simulink model "d_006"  (Simulink 9.3)
settings: Solver=ode45  StartTime=0.0  StopTime=10.0  RelTol=1e-3  EnableMultiTasking=on
settings Model: Creator=fmilano  LastModifiedBy=fmilano  ExtModeAutoUpdateStatusClock=off
settings DataIOCC: LimitDataPoints=on
settings OptimizationCC: BooleanDataType=off  InitFltsAndDblsToZero=on  LifeSpan=auto
settings DebuggingCC: SaveWithParameterizedLinksMsg=none  SignalResolutionControl=TryResolveAllWithWarning  MultiTaskDSMMsg=warning  MultiTaskCondExecSysMsg=none  FcnCallInpInsideContextMsg=error  SFUnexpectedBacktrackingDiag=error  SFNoUnconditionalDefaultTransitionDiag=error  SFExecutionAtInitializationDiag=warning  ArithmeticOperatorsInVariantConditions=error
settings HardwareCC: ProdBitPerPointer=64  ProdBitPerSizeT=64  ProdBitPerPtrDiffT=64  ProdLargestAtomicFloat=Float  ProdIntDivRoundTo=Zero  ProdEndianess=LittleEndian  ProdWordSize=64  ProdHWDeviceType=Intel->x86-64 (Windows64)  TargetUnknown=on
settings SFSimCC: SimUseLocalCustomCode=on
settings RTWCC: RTWUseLocalCustomCode=on
settings CodeAppCC: StateflowObjectComments=off
settings GRTTargetCC: TargetFcnLib=ansi_tfl_tmw.mat  TargetLangStandard=C99 (ISO)  CodeReplacementLibrary=ANSI_C  ParMdlRefBuildCompliant=off  CompOptLevelCompliant=off  CPPClassGenCompliant=off
settings ConfigComp: CovExternalEMLEnable=on

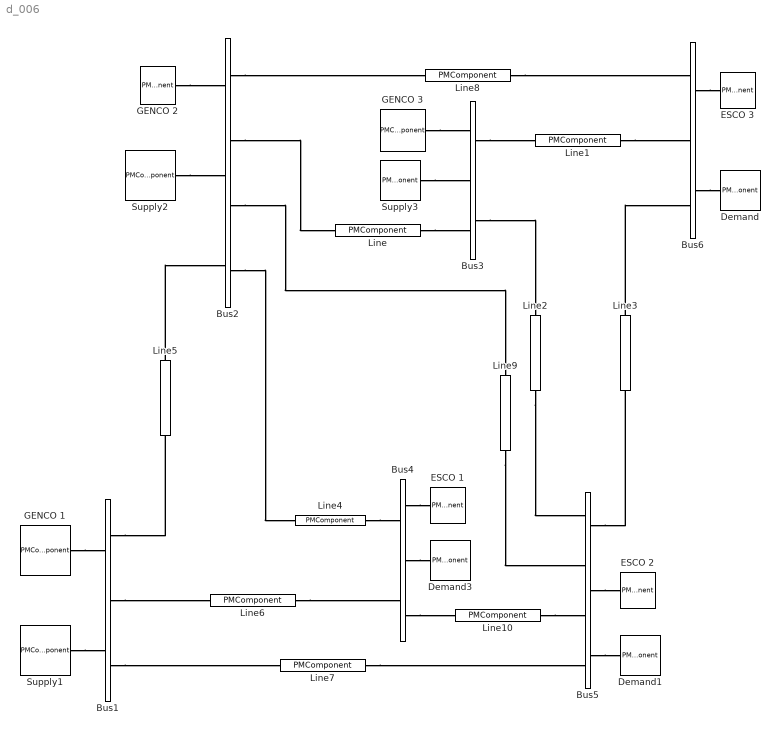
== system d_006 ==
  Bus1 : PMComponent  Tag=PSATblock  Description=Connection  PhysicalDomain=psatdomain  LeftPortType=p1  RightPortType=p1  LConnTagsString=__newl0|__newl1  RConnTagsString=__newr0|__newr1|__newr2  mask(Bus){in=2, out=3, p2q=400, p3_4q=[1.00   0.00], p5q=2, p6q=1}
      mask prompts: in "Number of inputs:"; out "Number of outputs:"; p2q "Voltage Rating [kV]"; p3_4q "Voltage initial guess [p.u.  rad]"; p5q "Area number"; p6q "Region number"
      mask help: Bus block.
      mask init:
      | fm_inout
      mask Callback p5q: fm_block
      mask Display: plot([0 1 1 0 0],[0 0 1 1 0])
  Bus2 : PMComponent  Tag=PSATblock  Description=Connection  PhysicalDomain=psatdomain  LeftPortType=p1  RightPortType=p1  LConnTagsString=__newl0|__newl1|__newl2  RConnTagsString=__newr0|__newr1|__newr2|__newr3  mask(Bus){in=3, out=4, p2q=400, p3_4q=[1.00   0.00], p5q=2, p6q=1}
      mask prompts: in "Number of inputs:"; out "Number of outputs:"; p2q "Voltage Rating [kV]"; p3_4q "Voltage initial guess [p.u.  rad]"; p5q "Area number"; p6q "Region number"
      mask help: Bus block.
      mask init:
      | fm_inout
      mask Callback p5q: fm_block
      mask Display: plot([0 1 1 0 0],[0 0 1 1 0])
  Bus3 : PMComponent  Tag=PSATblock  Description=Connection  PhysicalDomain=psatdomain  LeftPortType=p1  RightPortType=p1  LConnTagsString=__newl0|__newl1|__newl2  RConnTagsString=__newr0|__newr1  mask(Bus){in=3, out=2, p2q=400, p3_4q=[1.00   0.00], p5q=2, p6q=1}
      mask prompts: in "Number of inputs:"; out "Number of outputs:"; p2q "Voltage Rating [kV]"; p3_4q "Voltage initial guess [p.u.  rad]"; p5q "Area number"; p6q "Region number"
      mask help: Bus block.
      mask init:
      | fm_inout
      mask Callback p5q: fm_block
      mask Display: plot([0 1 1 0 0],[0 0 1 1 0])
  Bus4 : PMComponent  Tag=PSATblock  Description=Connection  PhysicalDomain=psatdomain  LeftPortType=p1  RightPortType=p1  LConnTagsString=__newl0|__newl1  RConnTagsString=__newr0|__newr1|__newr2  mask(Bus){in=2, out=3, p2q=400, p3_4q=[1.00   0.00], p5q=2, p6q=1}
      mask prompts: in "Number of inputs:"; out "Number of outputs:"; p2q "Voltage Rating [kV]"; p3_4q "Voltage initial guess [p.u.  rad]"; p5q "Area number"; p6q "Region number"
      mask help: Bus block.
      mask init:
      | fm_inout
      mask Callback p5q: fm_block
      mask Display: plot([0 1 1 0 0],[0 0 1 1 0])
  Bus5 : PMComponent  Tag=PSATblock  Description=Connection  PhysicalDomain=psatdomain  LeftPortType=p1  RightPortType=p1  LConnTagsString=__newl0|__newl1|__newl2|__newl3  RConnTagsString=__newr0|__newr1|__newr2  mask(Bus){in=4, out=3, p2q=400, p3_4q=[1.00   0.00], p5q=2, p6q=1}
      mask prompts: in "Number of inputs:"; out "Number of outputs:"; p2q "Voltage Rating [kV]"; p3_4q "Voltage initial guess [p.u.  rad]"; p5q "Area number"; p6q "Region number"
      mask help: Bus block.
      mask init:
      | fm_inout
      mask Callback p5q: fm_block
      mask Display: plot([0 1 1 0 0],[0 0 1 1 0])
  Bus6 : PMComponent  Tag=PSATblock  Description=Connection  PhysicalDomain=psatdomain  LeftPortType=p1  RightPortType=p1  LConnTagsString=__newl0|__newl1|__newl2  RConnTagsString=__newr0|__newr1  mask(Bus){in=3, out=2, p2q=400, p3_4q=[1.00   0.00], p5q=2, p6q=1}
      mask prompts: in "Number of inputs:"; out "Number of outputs:"; p2q "Voltage Rating [kV]"; p3_4q "Voltage initial guess [p.u.  rad]"; p5q "Area number"; p6q "Region number"
      mask help: Bus block.
      mask init:
      | fm_inout
      mask Callback p5q: fm_block
      mask Display: plot([0 1 1 0 0],[0 0 1 1 0])
  Demand : PMComponent  Tag=PSATblock  Description=OPF & CPF  PhysicalDomain=psatdomain  LeftPortType=p1  RightPortType=p1  LConnTagsString=__newl0  mask(Demand){p2q=100, p3q=0.2, p4q=0.66666*0.1, p5_6q=[0.2  0.00001], p8_9_10q=[0.00  9.5  0.00], p11_12_13q=[0.00  0.00  0.00], p14q=off, p15q=0, p16_17q=[0 0], out=0, p18q=on}
      mask prompts: p2q "Power Rating [MVA]"; p3q "Active Power [p.u.]"; p4q "Reactive Power [p.u.]"; p5_6q "Max and Min Power Demand [p.u.  p.u.]"; p8_9_10q "Cost = a + b*P + c*P^2 [$/h, $/MWh, $/(MW)^2 h]"; p11_12_13q "Cost = a + b*Q + c*Q^2 [$/h, $/MVArh, $/(MVAr)^2 h]"; p14q "Allow Unit Commitment"; p15q "Tie Breaking Cost [$/h]"; p16_17q "Up and down congestion costs [$/h $/h]"; out "Number of Output Signals"; p18q "Connected"
      mask help: This block defines a constant power load for bifurcation and market studies.
      mask init:
      | fm_inout;
      | [xs,ys]=fm_draw('$');
      mask TypeOptions out: 0 | 1
      mask Callback p18q: fm_block
      mask Display:
      | plot([ 1.0000    -0.5   -0.5  1],[ 0    0.866    -0.866    0])
      | color('blue')
      | plot(0.6*xs,0.6*ys)
  Demand1 : PMComponent  Tag=PSATblock  Description=OPF & CPF  PhysicalDomain=psatdomain  LeftPortType=p1  RightPortType=p1  LConnTagsString=__newl0  mask(Demand){p2q=100, p3q=0.1, p4q=0.7*0.1, p5_6q=[0.1  0.00001], p8_9_10q=[0.00  10.5  0.00], p11_12_13q=[0.00  0.00  0.00], p14q=off, p15q=0, p16_17q=[0 0], out=0, p18q=on}
      mask prompts: p2q "Power Rating [MVA]"; p3q "Active Power [p.u.]"; p4q "Reactive Power [p.u.]"; p5_6q "Max and Min Power Demand [p.u.  p.u.]"; p8_9_10q "Cost = a + b*P + c*P^2 [$/h, $/MWh, $/(MW)^2 h]"; p11_12_13q "Cost = a + b*Q + c*Q^2 [$/h, $/MVArh, $/(MVAr)^2 h]"; p14q "Allow Unit Commitment"; p15q "Tie Breaking Cost [$/h]"; p16_17q "Up and down congestion costs [$/h $/h]"; out "Number of Output Signals"; p18q "Connected"
      mask help: This block defines a constant power load for bifurcation and market studies.
      mask init:
      | fm_inout;
      | [xs,ys]=fm_draw('$');
      mask TypeOptions out: 0 | 1
      mask Callback p18q: fm_block
      mask Display:
      | plot([ 1.0000    -0.5   -0.5  1],[ 0    0.866    -0.866    0])
      | color('blue')
      | plot(0.6*xs,0.6*ys)
  Demand3 : PMComponent  Tag=PSATblock  Description=OPF & CPF  PhysicalDomain=psatdomain  LeftPortType=p1  RightPortType=p1  LConnTagsString=__newl0  mask(Demand){p2q=100, p3q=0.25, p4q=0.66666*0.25, p5_6q=[0.25  0.00001], p8_9_10q=[0.00  12  0.00], p11_12_13q=[0.00  0.00  0.00], p14q=off, p15q=0, p16_17q=[0 0], out=0, p18q=on}
      mask prompts: p2q "Power Rating [MVA]"; p3q "Active Power [p.u.]"; p4q "Reactive Power [p.u.]"; p5_6q "Max and Min Power Demand [p.u.  p.u.]"; p8_9_10q "Cost = a + b*P + c*P^2 [$/h, $/MWh, $/(MW)^2 h]"; p11_12_13q "Cost = a + b*Q + c*Q^2 [$/h, $/MVArh, $/(MVAr)^2 h]"; p14q "Allow Unit Commitment"; p15q "Tie Breaking Cost [$/h]"; p16_17q "Up and down congestion costs [$/h $/h]"; out "Number of Output Signals"; p18q "Connected"
      mask help: This block defines a constant power load for bifurcation and market studies.
      mask init:
      | fm_inout;
      | [xs,ys]=fm_draw('$');
      mask TypeOptions out: 0 | 1
      mask Callback p18q: fm_block
      mask Display:
      | plot([ 1.0000    -0.5   -0.5  1],[ 0    0.866    -0.866    0])
      | color('blue')
      | plot(0.6*xs,0.6*ys)
  ESCO 1 : PMComponent  Tag=PSATblock  Description=Power Flow  PhysicalDomain=psatdomain  LeftPortType=p1  RightPortType=p1  LConnTagsString=__newl0  mask(PQ){p2_3q=[100  400], p4_5q=[0.90  0.60], p6_7q=[1.1  0.9], p8q=off, p9q=on}
      mask prompts: p2_3q "Power and Voltage Ratings [MVA, kV]"; p4_5q "Active and Reactive Powers [p.u.  p.u.]"; p6_7q "Maximum and Minimum Allowable Voltage [p.u.   p.u.]"; p8q "Allow conversion to impendance for min & max voltage"; p9q "Connected"
      mask help:
      | This block defines a constant power load:
      |
      | P = Pcost.
      | Q = Qcost.
      mask Callback p8q: fm_block
      mask Callback p9q: fm_block
      mask Display: plot([1 -0.5 -0.5 1],[0 0.866 -0.866 0])
  ESCO 2 : PMComponent  Tag=PSATblock  Description=Power Flow  PhysicalDomain=psatdomain  LeftPortType=p1  RightPortType=p1  LConnTagsString=__newl0  mask(PQ){p2_3q=[100  400], p4_5q=[1.00  0.70], p6_7q=[1.1  0.9], p8q=off, p9q=on}
      mask prompts: p2_3q "Power and Voltage Ratings [MVA, kV]"; p4_5q "Active and Reactive Powers [p.u.  p.u.]"; p6_7q "Maximum and Minimum Allowable Voltage [p.u.   p.u.]"; p8q "Allow conversion to impendance for min & max voltage"; p9q "Connected"
      mask help:
      | This block defines a constant power load:
      |
      | P = Pcost.
      | Q = Qcost.
      mask Callback p8q: fm_block
      mask Callback p9q: fm_block
      mask Display: plot([1 -0.5 -0.5 1],[0 0.866 -0.866 0])
  ESCO 3 : PMComponent  Tag=PSATblock  Description=Power Flow  PhysicalDomain=psatdomain  LeftPortType=p1  RightPortType=p1  LConnTagsString=__newl0  mask(PQ){p2_3q=[100  400], p4_5q=[0.90  0.60], p6_7q=[1.1  0.9], p8q=off, p9q=on}
      mask prompts: p2_3q "Power and Voltage Ratings [MVA, kV]"; p4_5q "Active and Reactive Powers [p.u.  p.u.]"; p6_7q "Maximum and Minimum Allowable Voltage [p.u.   p.u.]"; p8q "Allow conversion to impendance for min & max voltage"; p9q "Connected"
      mask help:
      | This block defines a constant power load:
      |
      | P = Pcost.
      | Q = Qcost.
      mask Callback p8q: fm_block
      mask Callback p9q: fm_block
      mask Display: plot([1 -0.5 -0.5 1],[0 0.866 -0.866 0])
  GENCO 1 : PMComponent  Tag=PSATblock  Description=Power Flow  PhysicalDomain=psatdomain  LeftPortType=p1  RightPortType=p1  RConnTagsString=__newr0  mask(PV){p2_3q=[100  400], p4q=0.9, p5q=1.05, p6_7q=[1.5  -1.5], p8_9q=[1.1  0.9], p10q=1, p11q=on}
      mask prompts: p2_3q "Power and Voltage Ratings [MVA, kV]"; p4q "Active Power [p.u.]"; p5q "Voltage Magnitude [p.u.]"; p6_7q "Qmax & Qmin [p.u.  p.u.]"; p8_9q "Vmax & Vmin [p.u.  p.u.]"; p10q "Loss Participation Factor"; p11q "Connected"
      mask help:
      | This block defines a PV bus for load flow studies:
      |
      | P = Pcost.
      | V = Vdes.
      mask init:
      | [x,y] = fm_draw('circle');
      | [xp,yp] = fm_draw('P');
      mask Callback p11q: fm_block
      mask Display:
      | plot(x,y)
      | color('blue')
      | plot(0.3*xp-0.35,0.6*yp,[0.1 0.3 0.5],[0.3 -0.3 0.3])
  GENCO 2 : PMComponent  Tag=PSATblock  Description=Power Flow  PhysicalDomain=psatdomain  LeftPortType=p1  RightPortType=p1  RConnTagsString=__newr0  mask(SW){p2_3q=[100  400], p4q=1.05, p5q=0.00, p6_7q=[1.5  -1.5], p8_9q=[1.1  0.9], p10q=1.4, p11q=1, p12q=on, p13q=on}
      mask prompts: p2_3q "Power and Voltage Ratings [MVA, kV]"; p4q "Voltage Magnitude [p.u.]"; p5q "Reference Phase Angle [rad]"; p6_7q "Qmax and Qmin [p.u.  p.u.]"; p8_9q "Vmax and Vmin  [p.u.  p.u.]"; p10q "Active Power Guess [p.u.]"; p11q "Loss Participation Factor"; p12q "Reference bus"; p13q "Connected"
      mask help:
      | This block defines a V-theta bus:
      |
      | V = V_des
      | theta = theta_des
      mask init:
      | [x,y] = fm_draw('circle');
      | [xt,yt] = fm_draw('theta');
      mask Callback p12q: fm_block
      mask Callback p13q: fm_block
      mask Display: plot([0 1 1 0 0],[0 0 1 1 0]), color('blue'), plot([0 1],[0 1],[0 1],[1 0],[0.5 1 0.5 0 0.5],[0 0.5 1 0.5 0])
  GENCO 3 : PMComponent  Tag=PSATblock  Description=Power Flow  PhysicalDomain=psatdomain  LeftPortType=p1  RightPortType=p1  RConnTagsString=__newr0  mask(PV){p2_3q=[100  400], p4q=0.6, p5q=1.05, p6_7q=[1.5  -1.5], p8_9q=[1.1  0.9], p10q=1, p11q=on}
      mask prompts: p2_3q "Power and Voltage Ratings [MVA, kV]"; p4q "Active Power [p.u.]"; p5q "Voltage Magnitude [p.u.]"; p6_7q "Qmax & Qmin [p.u.  p.u.]"; p8_9q "Vmax & Vmin [p.u.  p.u.]"; p10q "Loss Participation Factor"; p11q "Connected"
      mask help:
      | This block defines a PV bus for load flow studies:
      |
      | P = Pcost.
      | V = Vdes.
      mask init:
      | [x,y] = fm_draw('circle');
      | [xp,yp] = fm_draw('P');
      mask Callback p11q: fm_block
      mask Display:
      | plot(x,y)
      | color('blue')
      | plot(0.3*xp-0.35,0.6*yp,[0.1 0.3 0.5],[0.3 -0.3 0.3])
  Line : PMComponent  Tag=PSATblock  Description=Power Flow  PhysicalDomain=psatdomain  LeftPortType=p1  RightPortType=p1  LConnTagsString=__newl0  RConnTagsString=__newr0  mask(Line){p3_4_5q=[100  400  60], p6q=0, p8q=0.05, p9q=0.25, p10q=0.06, p13_14_15q=[0.3082  0.0  0.0], p16q=on}
      mask prompts: p3_4_5q "Power, Voltage and Frequency Ratings [MVA, kV, Hz]"; p6q "Length of line [km] (0 for p.u. parameters)"; p8q "Resistance [p.u. (Ohms/km)]"; p9q "Reactance [p.u. (H/km)]"; p10q "Susceptance [p.u. (F/km)]"; p13_14_15q "Imax, Pmax and Smax [p.u., p.u., p.u.]"; p16q "Connected"
      mask help: This block defines a pi model for a tree phase line.
      mask init:
      | [xp,yp] = fm_draw('pi');
      mask Callback p16q: fm_block
      mask Display:
      | plot([-1  1  1 -1 -1],[-0.2 -0.2 0.2 0.2 -0.2])
      | color('blue')
      | plot(0.35*xp,0.2*yp)
  Line1 : PMComponent  Tag=PSATblock  Description=Power Flow  PhysicalDomain=psatdomain  LeftPortType=p1  RightPortType=p1  LConnTagsString=__newl0  RConnTagsString=__newr0  mask(Line){p3_4_5q=[100  400  60], p6q=0, p8q=0.02, p9q=0.10, p10q=0.02, p13_14_15q=[1.3973  0.0  0.0], p16q=on}
      mask prompts: p3_4_5q "Power, Voltage and Frequency Ratings [MVA, kV, Hz]"; p6q "Length of line [km] (0 for p.u. parameters)"; p8q "Resistance [p.u. (Ohms/km)]"; p9q "Reactance [p.u. (H/km)]"; p10q "Susceptance [p.u. (F/km)]"; p13_14_15q "Imax, Pmax and Smax [p.u., p.u., p.u.]"; p16q "Connected"
      mask help: This block defines a pi model for a tree phase line.
      mask init:
      | [xp,yp] = fm_draw('pi');
      mask Callback p16q: fm_block
      mask Display:
      | plot([-1  1  1 -1 -1],[-0.2 -0.2 0.2 0.2 -0.2])
      | color('blue')
      | plot(0.35*xp,0.2*yp)
  Line10 : PMComponent  Tag=PSATblock  Description=Power Flow  PhysicalDomain=psatdomain  LeftPortType=p1  RightPortType=p1  LConnTagsString=__newl0  RConnTagsString=__newr0  mask(Line){p3_4_5q=[100  400  60], p6q=0, p8q=0.2, p9q=0.4, p10q=0.08, p13_14_15q=[0.1796  0.0  0.0], p16q=on}
      mask prompts: p3_4_5q "Power, Voltage and Frequency Ratings [MVA, kV, Hz]"; p6q "Length of line [km] (0 for p.u. parameters)"; p8q "Resistance [p.u. (Ohms/km)]"; p9q "Reactance [p.u. (H/km)]"; p10q "Susceptance [p.u. (F/km)]"; p13_14_15q "Imax, Pmax and Smax [p.u., p.u., p.u.]"; p16q "Connected"
      mask help: This block defines a pi model for a tree phase line.
      mask init:
      | [xp,yp] = fm_draw('pi');
      mask Callback p16q: fm_block
      mask Display:
      | plot([-1  1  1 -1 -1],[-0.2 -0.2 0.2 0.2 -0.2])
      | color('blue')
      | plot(0.35*xp,0.2*yp)
  Line2 : PMComponent  Tag=PSATblock  Description=Power Flow  PhysicalDomain=psatdomain  LeftPortType=p1  RightPortType=p1  LConnTagsString=__newl0  RConnTagsString=__newr0  mask(Line){p3_4_5q=[100  400  60], p6q=0, p8q=0.12, p9q=0.26, p10q=0.05, p13_14_15q=[0.6585  0.0  0.0], p16q=on}
      mask prompts: p3_4_5q "Power, Voltage and Frequency Ratings [MVA, kV, Hz]"; p6q "Length of line [km] (0 for p.u. parameters)"; p8q "Resistance [p.u. (Ohms/km)]"; p9q "Reactance [p.u. (H/km)]"; p10q "Susceptance [p.u. (F/km)]"; p13_14_15q "Imax, Pmax and Smax [p.u., p.u., p.u.]"; p16q "Connected"
      mask help: This block defines a pi model for a tree phase line.
      mask init:
      | [xp,yp] = fm_draw('pi');
      mask Callback p16q: fm_block
      mask Display:
      | plot([-1  1  1 -1 -1],[-0.2 -0.2 0.2 0.2 -0.2])
      | color('blue')
      | plot(0.35*xp,0.2*yp)
  Line3 : PMComponent  Tag=PSATblock  Description=Power Flow  PhysicalDomain=psatdomain  LeftPortType=p1  RightPortType=p1  LConnTagsString=__newl0  RConnTagsString=__newr0  mask(Line){p3_4_5q=[100  400  60], p6q=0, p8q=0.1, p9q=0.30, p10q=0.06, p13_14_15q=[0.2  0.0  0.0], p16q=on}
      mask prompts: p3_4_5q "Power, Voltage and Frequency Ratings [MVA, kV, Hz]"; p6q "Length of line [km] (0 for p.u. parameters)"; p8q "Resistance [p.u. (Ohms/km)]"; p9q "Reactance [p.u. (H/km)]"; p10q "Susceptance [p.u. (F/km)]"; p13_14_15q "Imax, Pmax and Smax [p.u., p.u., p.u.]"; p16q "Connected"
      mask help: This block defines a pi model for a tree phase line.
      mask init:
      | [xp,yp] = fm_draw('pi');
      mask Callback p16q: fm_block
      mask Display:
      | plot([-1  1  1 -1 -1],[-0.2 -0.2 0.2 0.2 -0.2])
      | color('blue')
      | plot(0.35*xp,0.2*yp)
  Line4 : PMComponent  Tag=PSATblock  Description=Power Flow  PhysicalDomain=psatdomain  LeftPortType=p1  RightPortType=p1  LConnTagsString=__newl0  RConnTagsString=__newr0  mask(Line){p3_4_5q=[100  400  60], p6q=0, p8q=0.05, p9q=0.10, p10q=0.02, p13_14_15q=[1.3740  0.0  0.0], p16q=on}
      mask prompts: p3_4_5q "Power, Voltage and Frequency Ratings [MVA, kV, Hz]"; p6q "Length of line [km] (0 for p.u. parameters)"; p8q "Resistance [p.u. (Ohms/km)]"; p9q "Reactance [p.u. (H/km)]"; p10q "Susceptance [p.u. (F/km)]"; p13_14_15q "Imax, Pmax and Smax [p.u., p.u., p.u.]"; p16q "Connected"
      mask help: This block defines a pi model for a tree phase line.
      mask init:
      | [xp,yp] = fm_draw('pi');
      mask Callback p16q: fm_block
      mask Display:
      | plot([-1  1  1 -1 -1],[-0.2 -0.2 0.2 0.2 -0.2])
      | color('blue')
      | plot(0.35*xp,0.2*yp)
  Line5 : PMComponent  Tag=PSATblock  Description=Power Flow  PhysicalDomain=psatdomain  LeftPortType=p1  RightPortType=p1  LConnTagsString=__newl0  RConnTagsString=__newr0  mask(Line){p3_4_5q=[100  400  60], p6q=0, p8q=0.1, p9q=0.2, p10q=0.04, p13_14_15q=[0.2591  0.0  0.0], p16q=on}
      mask prompts: p3_4_5q "Power, Voltage and Frequency Ratings [MVA, kV, Hz]"; p6q "Length of line [km] (0 for p.u. parameters)"; p8q "Resistance [p.u. (Ohms/km)]"; p9q "Reactance [p.u. (H/km)]"; p10q "Susceptance [p.u. (F/km)]"; p13_14_15q "Imax, Pmax and Smax [p.u., p.u., p.u.]"; p16q "Connected"
      mask help: This block defines a pi model for a tree phase line.
      mask init:
      | [xp,yp] = fm_draw('pi');
      mask Callback p16q: fm_block
      mask Display:
      | plot([-1  1  1 -1 -1],[-0.2 -0.2 0.2 0.2 -0.2])
      | color('blue')
      | plot(0.35*xp,0.2*yp)
  Line6 : PMComponent  Tag=PSATblock  Description=Power Flow  PhysicalDomain=psatdomain  LeftPortType=p1  RightPortType=p1  LConnTagsString=__newl0  RConnTagsString=__newr0  mask(Line){p3_4_5q=[100  400  60], p6q=0, p8q=0.05, p9q=0.20, p10q=0.04, p13_14_15q=[0.9193  0.0  0.0], p16q=on}
      mask prompts: p3_4_5q "Power, Voltage and Frequency Ratings [MVA, kV, Hz]"; p6q "Length of line [km] (0 for p.u. parameters)"; p8q "Resistance [p.u. (Ohms/km)]"; p9q "Reactance [p.u. (H/km)]"; p10q "Susceptance [p.u. (F/km)]"; p13_14_15q "Imax, Pmax and Smax [p.u., p.u., p.u.]"; p16q "Connected"
      mask help: This block defines a pi model for a tree phase line.
      mask init:
      | [xp,yp] = fm_draw('pi');
      mask Callback p16q: fm_block
      mask Display:
      | plot([-1  1  1 -1 -1],[-0.2 -0.2 0.2 0.2 -0.2])
      | color('blue')
      | plot(0.35*xp,0.2*yp)
  Line7 : PMComponent  Tag=PSATblock  Description=Power Flow  PhysicalDomain=psatdomain  LeftPortType=p1  RightPortType=p1  LConnTagsString=__newl0  RConnTagsString=__newr0  mask(Line){p3_4_5q=[100  400  60], p6q=0, p8q=0.08, p9q=0.30, p10q=0.06, p13_14_15q=[0.8478  0.0  0.0], p16q=on}
      mask prompts: p3_4_5q "Power, Voltage and Frequency Ratings [MVA, kV, Hz]"; p6q "Length of line [km] (0 for p.u. parameters)"; p8q "Resistance [p.u. (Ohms/km)]"; p9q "Reactance [p.u. (H/km)]"; p10q "Susceptance [p.u. (F/km)]"; p13_14_15q "Imax, Pmax and Smax [p.u., p.u., p.u.]"; p16q "Connected"
      mask help: This block defines a pi model for a tree phase line.
      mask init:
      | [xp,yp] = fm_draw('pi');
      mask Callback p16q: fm_block
      mask Display:
      | plot([-1  1  1 -1 -1],[-0.2 -0.2 0.2 0.2 -0.2])
      | color('blue')
      | plot(0.35*xp,0.2*yp)
  Line8 : PMComponent  Tag=PSATblock  Description=Power Flow  PhysicalDomain=psatdomain  LeftPortType=p1  RightPortType=p1  LConnTagsString=__newl0  RConnTagsString=__newr0  mask(Line){p3_4_5q=[100  400  60], p6q=0, p8q=0.07, p9q=0.2, p10q=0.05, p13_14_15q=[0.9147  0.0  0.0], p16q=on}
      mask prompts: p3_4_5q "Power, Voltage and Frequency Ratings [MVA, kV, Hz]"; p6q "Length of line [km] (0 for p.u. parameters)"; p8q "Resistance [p.u. (Ohms/km)]"; p9q "Reactance [p.u. (H/km)]"; p10q "Susceptance [p.u. (F/km)]"; p13_14_15q "Imax, Pmax and Smax [p.u., p.u., p.u.]"; p16q "Connected"
      mask help: This block defines a pi model for a tree phase line.
      mask init:
      | [xp,yp] = fm_draw('pi');
      mask Callback p16q: fm_block
      mask Display:
      | plot([-1  1  1 -1 -1],[-0.2 -0.2 0.2 0.2 -0.2])
      | color('blue')
      | plot(0.35*xp,0.2*yp)
  Line9 : PMComponent  Tag=PSATblock  Description=Power Flow  PhysicalDomain=psatdomain  LeftPortType=p1  RightPortType=p1  LConnTagsString=__newl0  RConnTagsString=__newr0  mask(Line){p3_4_5q=[100  400  60], p6q=0, p8q=0.1, p9q=0.3, p10q=0.04, p13_14_15q=[0.7114  0.0  0.0], p16q=on}
      mask prompts: p3_4_5q "Power, Voltage and Frequency Ratings [MVA, kV, Hz]"; p6q "Length of line [km] (0 for p.u. parameters)"; p8q "Resistance [p.u. (Ohms/km)]"; p9q "Reactance [p.u. (H/km)]"; p10q "Susceptance [p.u. (F/km)]"; p13_14_15q "Imax, Pmax and Smax [p.u., p.u., p.u.]"; p16q "Connected"
      mask help: This block defines a pi model for a tree phase line.
      mask init:
      | [xp,yp] = fm_draw('pi');
      mask Callback p16q: fm_block
      mask Display:
      | plot([-1  1  1 -1 -1],[-0.2 -0.2 0.2 0.2 -0.2])
      | color('blue')
      | plot(0.35*xp,0.2*yp)
  Supply1 : PMComponent  Tag=PSATblock  Description=OPF & CPF  PhysicalDomain=psatdomain  LeftPortType=p1  RightPortType=p1  RConnTagsString=__newr0  mask(Supply){p2q=100, p3q=0.2, p4_5q=[0.2  0.00001], p7_8_9q=[0.00  9.70  0.00], p10_11_12q=[0.00  0.00  0.00], p13q=off, p14q=0, p15q=1, p16_17q=[1.5  -1.5], p18_19q=[0 0], in=0, p20q=on}
      mask prompts: p2q "Power Rating [MVA]"; p3q "Active Power [p.u.]"; p4_5q "Max and Min Power Supply [p.u.  p.u.]"; p7_8_9q "Cost = a + b*P + c*P^2 [$/h, $/MWh, $/(MW)^2 h]"; p10_11_12q "Cost = a + b*Q + c*Q^2 [$/h, $/MVArh, $/(MVAr)^2 h]"; p13q "Allow Unit Commitment"; p14q "Tie Breaking Cost [$/h]"; p15q "Loss participation factor"; p16_17q "Reactive power limits Qmax and Qmin [p.u. p.u.]"; p18_19q "Up and down congestion costs [$/h $/h]"; in "Number of Input Signals"; p20q "Connected"
      mask help: This block defines a PV bus for bifurcation and market studies:
      mask init:
      | fm_inout;
      | [x,y] = fm_draw('circle');
      | [xs,ys] = fm_draw('$');
      mask TypeOptions in: 0 | 1 | 2
      mask Callback p20q: fm_block
      mask Display:
      | plot(x,y)
      | color('blue')
      | plot(xs,ys)
  Supply2 : PMComponent  Tag=PSATblock  Description=OPF & CPF  PhysicalDomain=psatdomain  LeftPortType=p1  RightPortType=p1  RConnTagsString=__newr0  mask(Supply){p2q=100, p3q=0.25, p4_5q=[0.25 0.00001], p7_8_9q=[0.00  8.80  0.00], p10_11_12q=[0.00  0.00  0.00], p13q=off, p14q=0, p15q=1, p16_17q=[1.5  -1.5], p18_19q=[0 0], in=0, p20q=on}
      mask prompts: p2q "Power Rating [MVA]"; p3q "Active Power [p.u.]"; p4_5q "Max and Min Power Supply [p.u.  p.u.]"; p7_8_9q "Cost = a + b*P + c*P^2 [$/h, $/MWh, $/(MW)^2 h]"; p10_11_12q "Cost = a + b*Q + c*Q^2 [$/h, $/MVArh, $/(MVAr)^2 h]"; p13q "Allow Unit Commitment"; p14q "Tie Breaking Cost [$/h]"; p15q "Loss participation factor"; p16_17q "Reactive power limits Qmax and Qmin [p.u. p.u.]"; p18_19q "Up and down congestion costs [$/h $/h]"; in "Number of Input Signals"; p20q "Connected"
      mask help: This block defines a PV bus for bifurcation and market studies:
      mask init:
      | fm_inout;
      | [x,y] = fm_draw('circle');
      | [xs,ys] = fm_draw('$');
      mask TypeOptions in: 0 | 1 | 2
      mask Callback p20q: fm_block
      mask Display:
      | plot(x,y)
      | color('blue')
      | plot(xs,ys)
  Supply3 : PMComponent  Tag=PSATblock  Description=OPF & CPF  PhysicalDomain=psatdomain  LeftPortType=p1  RightPortType=p1  RConnTagsString=__newr0  mask(Supply){p2q=100, p3q=0.2, p4_5q=[0.2  0.00001], p7_8_9q=[0.00  7.0  0.00], p10_11_12q=[0.00  0.00  0.00], p13q=off, p14q=0, p15q=1, p16_17q=[1.5  -1.5], p18_19q=[0 0], in=0, p20q=on}
      mask prompts: p2q "Power Rating [MVA]"; p3q "Active Power [p.u.]"; p4_5q "Max and Min Power Supply [p.u.  p.u.]"; p7_8_9q "Cost = a + b*P + c*P^2 [$/h, $/MWh, $/(MW)^2 h]"; p10_11_12q "Cost = a + b*Q + c*Q^2 [$/h, $/MVArh, $/(MVAr)^2 h]"; p13q "Allow Unit Commitment"; p14q "Tie Breaking Cost [$/h]"; p15q "Loss participation factor"; p16_17q "Reactive power limits Qmax and Qmin [p.u. p.u.]"; p18_19q "Up and down congestion costs [$/h $/h]"; in "Number of Input Signals"; p20q "Connected"
      mask help: This block defines a PV bus for bifurcation and market studies:
      mask init:
      | fm_inout;
      | [x,y] = fm_draw('circle');
      | [xs,ys] = fm_draw('$');
      mask TypeOptions in: 0 | 1 | 2
      mask Callback p20q: fm_block
      mask Display:
      | plot(x,y)
      | color('blue')
      | plot(xs,ys)
  connections:
  Line7/RConn1 -- Bus5/LConn4
  Bus1/RConn3 -- Line7/LConn1
  Bus2/RConn3 -- Line9/LConn1
  Line4/RConn1 -- Bus4/LConn1
  Bus2/RConn4 -- Line4/LConn1
  Line6/RConn1 -- Bus4/LConn2
  Supply3/RConn1 -- Bus3/LConn2
  Line/RConn1 -- Bus3/LConn3
  Supply2/RConn1 -- Bus2/LConn2
  Supply1/RConn1 -- Bus1/LConn2
  Bus4/RConn2 -- Demand3/LConn1
  Bus4/RConn3 -- Line10/LConn1
  Bus6/RConn2 -- Demand/LConn1
  Bus5/RConn3 -- Demand1/LConn1
  GENCO 1/RConn1 -- Bus1/LConn1
  GENCO 2/RConn1 -- Bus2/LConn1
  Bus6/RConn1 -- ESCO 3/LConn1
  Line10/RConn1 -- Bus5/LConn3
  Bus4/RConn1 -- ESCO 1/LConn1
  Line9/RConn1 -- Bus5/LConn2
  Line8/RConn1 -- Bus6/LConn1
  Line1/RConn1 -- Bus6/LConn2
  Line3/RConn1 -- Bus6/LConn3
  Bus2/RConn2 -- Line/LConn1
  Bus2/RConn1 -- Line8/LConn1
  Bus1/RConn2 -- Line6/LConn1
  Bus1/RConn1 -- Line5/LConn1
  Bus5/RConn1 -- Line3/LConn1
  Line2/RConn1 -- Bus5/LConn1
  Bus3/RConn2 -- Line2/LConn1
  Bus3/RConn1 -- Line1/LConn1
  Bus5/RConn2 -- ESCO 2/LConn1
  GENCO 3/RConn1 -- Bus3/LConn1
  Line5/RConn1 -- Bus2/LConn3
